simulink model "LearnRateLimiter_Model_11182014"  (R2014b)
settings: Solver=ode45  StartTime=0.0  StopTime=10.0  RelTol=1e-3
libraries: simulink x5, simulink_extras x3
settings Model: Creator=RaymondSutjiono  LastModifiedBy=RaymondSutjiono

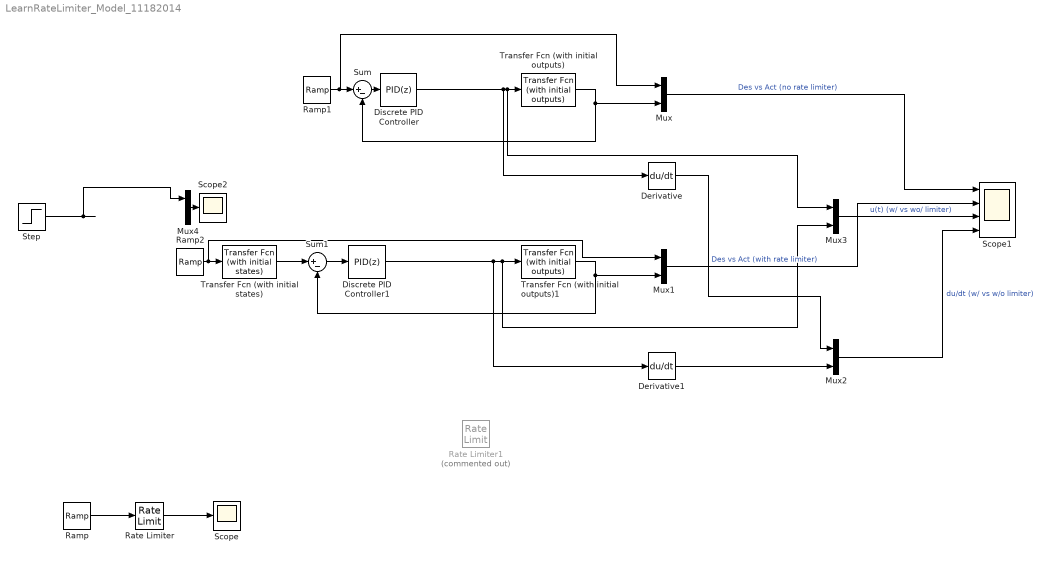
== system LearnRateLimiter_Model_11182014 ==
  Derivative : Derivative
  Derivative1 : Derivative
  Discrete PID Controller : simulink/Continuous/PID Controller  Controller=PID  TimeDomain=Discrete-time  SampleTime=0.005  IntegratorMethod=Forward Euler  FilterMethod=Forward Euler  Form=Parallel  P=20  I=2  D=0  N=100  InitialConditionSource=internal  InitialConditionForIntegrator=0  InitialConditionForFilter=0  ExternalReset=none  LimitOutput=off  UpperSaturationLimit=inf  LowerSaturationLimit=-inf  LinearizeAsGain=off  AntiWindupMode=none  Kb=1  TrackingMode=off  Kt=1  PParamMin=[]  PParamMax=[]  IParamMin=[]  IParamMax=[]  DParamMin=[]  DParamMax=[]  NParamMin=[]  NParamMax=[]  KbParamMin=[]  KbParamMax=[]  KtParamMin=[]  KtParamMax=[]  POutMin=[]  POutMax=[]  IOutMin=[]  IOutMax=[]  DOutMin=[]  DOutMax=[]  NOutMin=[]  NOutMax=[]  KbOutMin=[]  KbOutMax=[]  KtOutMin=[]  KtOutMax=[]  IntegratorOutMin=[]  IntegratorOutMax=[]  FilterOutMin=[]  FilterOutMax=[]  SumOutMin=[]  SumOutMax=[]  SumI1OutMin=[]  SumI1OutMax=[]  SumI2OutMin=[]  SumI2OutMax=[]  SumI3OutMin=[]  SumI3OutMax=[]  SumDOutMin=[]  SumDOutMax=[]  SaturationOutMin=[]  SaturationOutMax=[]  IntegratorContinuousStateAttributes=''  IntegratorStateMustResolveToSignalObject=off  IntegratorRTWStateStorageClass=Auto  FilterContinuousStateAttributes=''  FilterStateMustResolveToSignalObject=off  FilterRTWStateStorageClass=Auto  DifferentiatorICPrevScaledInput=0  DifferentiatorOutMin=[]  DifferentiatorOutMax=[]  UseFilter=on
  Discrete PID Controller1 : simulink/Continuous/PID Controller  Controller=PID  TimeDomain=Discrete-time  SampleTime=0.005  IntegratorMethod=Forward Euler  FilterMethod=Forward Euler  Form=Parallel  P=100  I=2  D=0  N=100  InitialConditionSource=internal  InitialConditionForIntegrator=0  InitialConditionForFilter=0  ExternalReset=none  LimitOutput=off  UpperSaturationLimit=inf  LowerSaturationLimit=-inf  LinearizeAsGain=off  AntiWindupMode=none  Kb=1  TrackingMode=off  Kt=1  PParamMin=[]  PParamMax=[]  IParamMin=[]  IParamMax=[]  DParamMin=[]  DParamMax=[]  NParamMin=[]  NParamMax=[]  KbParamMin=[]  KbParamMax=[]  KtParamMin=[]  KtParamMax=[]  POutMin=[]  POutMax=[]  IOutMin=[]  IOutMax=[]  DOutMin=[]  DOutMax=[]  NOutMin=[]  NOutMax=[]  KbOutMin=[]  KbOutMax=[]  KtOutMin=[]  KtOutMax=[]  IntegratorOutMin=[]  IntegratorOutMax=[]  FilterOutMin=[]  FilterOutMax=[]  SumOutMin=[]  SumOutMax=[]  SumI1OutMin=[]  SumI1OutMax=[]  SumI2OutMin=[]  SumI2OutMax=[]  SumI3OutMin=[]  SumI3OutMax=[]  SumDOutMin=[]  SumDOutMax=[]  SaturationOutMin=[]  SaturationOutMax=[]  IntegratorContinuousStateAttributes=''  IntegratorStateMustResolveToSignalObject=off  IntegratorRTWStateStorageClass=Auto  FilterContinuousStateAttributes=''  FilterStateMustResolveToSignalObject=off  FilterRTWStateStorageClass=Auto  DifferentiatorICPrevScaledInput=0  DifferentiatorOutMin=[]  DifferentiatorOutMax=[]  UseFilter=on
  Mux{,1..4} (5 alike) : Mux  Inputs=2
  Ramp : simulink/Sources/Ramp  slope=100  start=2  X0=0
  Ramp1 : simulink/Sources/Ramp  slope=10  start=2  X0=0
  Ramp2 : simulink/Sources/Ramp  slope=10  start=2  X0=0
  Rate Limiter : RateLimiter  RisingSlewLimit=90  SampleTimeMode=inherited
  Rate Limiter1 : RateLimiter  Commented=on  RisingSlewLimit=100  FallingSlewLimit=-100  SampleTimeMode=inherited
  Scope : Scope
  Scope1 : Scope  NumInputPorts=4
      settings: YMin=-5~-5~-5~-100  YMax=5~5~5~100
  Scope2 : Scope
      settings: SaveName=ScopeData2
  Step : Step  SampleTime=0
  Sum : Sum  Inputs=|+-
  Sum1 : Sum  Inputs=|+-
  Transfer Fcn (with initial outputs) : simulink_extras/Additional Linear/Transfer Fcn (with initial outputs)  N=[1]  D="[1  1]"  Y0=0  U0=0
  Transfer Fcn (with initial outputs)1 : simulink_extras/Additional Linear/Transfer Fcn (with initial outputs)  N=[1]  D="[1  1]"  Y0=0  U0=0
  Transfer Fcn (with initial states) : simulink_extras/Additional Linear/Transfer Fcn (with initial states)  N=5  D="[1  5]"  X0=0
  wires:
  Ramp/1 -> Rate Limiter/1
  Rate Limiter/1 -> Scope/1
  Transfer Fcn (with initial outputs)/1 -> Mux/2, Sum/2
  Sum/1 -> Discrete PID Controller/1
  Ramp1/1 -> Mux/1, Sum/1
  Mux/1 -> Scope1/1  "Des vs Act (no rate limiter)"
  Derivative/1 -> Mux2/1
  Transfer Fcn (with initial outputs)1/1 -> Mux1/2, Sum1/2
  Sum1/1 -> Discrete PID Controller1/1
  Ramp2/1 -> Mux1/1, Transfer Fcn (with initial states)/1
  Mux1/1 -> Scope1/2  "Des vs Act (with rate limiter)"
  Derivative1/1 -> Mux2/2
  Discrete PID Controller1/1 -> Mux3/2, Transfer Fcn (with initial outputs)1/1, Derivative1/1
  Mux3/1 -> Scope1/3  "u(t) (w/ vs wo/ limiter)"
  Mux2/1 -> Scope1/4  "du/dt (w/ vs w/o limiter)"
  Step/1 -> Mux4/1
  ? -> Mux4/2
  Mux4/1 -> Scope2/1
  Discrete PID Controller/1 -> Derivative/1, Mux3/1, Transfer Fcn (with initial outputs)/1
  Transfer Fcn (with initial states)/1 -> Sum1/1
